simulink model "duc_model"  (R2023b)
settings: Solver=VariableStepDiscrete  StartTime=0.0  StopTime=DUC_LINEUP_param.endTime  RelTol=1e-3  EnableMultiTasking=on
PreLoadFcn:
  | % Run the setup script when the model is opened
  | setup_duc_model;
InitFcn:
  | % Run the setup script again just before the
  | % model is run, so that any updates made
  | % after opening are applied.
  | 
  | setup_duc_model;
StopFcn:
  | DUC_Output_analysis
values from neighbouring files (symbols this model uses):
  DUC_CM_multiplication_factor = 1    [setup_duc_model.m]
  DUC_CM_NCO_phase = [0 0 0 0]    [setup_duc_model.m]
  DUC_CM_NCO_sync = [0 0 0 0]    [setup_duc_model.m]
  DUC_CM_number_of_bits_to_shift_left = 0    [setup_duc_model.m]
undefined symbols (not defined in the file or in its folder): AdvDSPBChannelOutDisplay, dspba_ChannelInVis, dspba_ChannelOutVis, dspba_internal_get_channel_ports, DUC_LINEUP_param, latency, value
libraries: DSPBABase x17, DSPBAPrim x14, DSPBAFilters x6, simulink x4, DSPBAWaveformSynth x2, DSPBAModelBus x2
Description:
  | DSP Builder Advanced Template for Template Design implementing ModelIP designs
settings Model: Creator=mjervis  LastModifiedBy=5g
settings SolverCC: AlgebraicLoopSolver=TrustRegion
settings DataIOCC: LimitDataPoints=on  SaveFormat=Array  SignalLoggingSaveFormat=ModelDataLogs  ReturnWorkspaceOutputs=off
settings OptimizationCC: ExpressionDepthLimit=2147483647  LifeSpan=inf
settings DebuggingCC: UnderspecifiedInitializationDetection=Classic  MergeDetectMultiDrivingBlocksExec=none  SolverPrmCheckMsg=warning  InheritedTsInSrcMsg=none  IntegerOverflowMsg=none  FcnCallInpInsideContextMsg=warning  UnconnectedInputMsg=warning  UnconnectedOutputMsg=warning  UnconnectedLineMsg=warning  StateNameClashWarn=warning  SFUnexpectedBacktrackingDiag=warning  SFNoUnconditionalDefaultTransitionDiag=warning  SFExecutionAtInitializationDiag=none  IntegerSaturationMsg=none  ArithmeticOperatorsInVariantConditions=warning
settings HardwareCC: ProdBitPerPointer=32  ProdBitPerSizeT=32  ProdBitPerPtrDiffT=32  ProdLargestAtomicFloat=None  ProdIntDivRoundTo=Undefined  ProdEndianess=Unspecified  ProdWordSize=32  ProdHWDeviceType=32-bit Generic
settings ModelReferenceCC: EnableRefExpFcnMdlSchedulingChecks=on  PropagateSignalLabelsOutOfModel=off
settings SFSimCC: SimUseLocalCustomCode=off  CustomCodeUndefinedFunction=UseInterfaceOnly
settings RTWCC: RTWUseLocalCustomCode=off  DLArmComputeVersion=19.05
settings CodeAppCC: StateflowObjectComments=on
settings GRTTargetCC: TargetLangStandard=C89/C90 (ANSI)  CombineOutputUpdateFcns=off  GRTInterface=on
settings ConfigComp: CovMetricSettings=dw  CovSaveCumulativeToWorkspaceVar=on  CovSaveSingleToWorkspaceVar=on  CovExternalEMLEnable=off

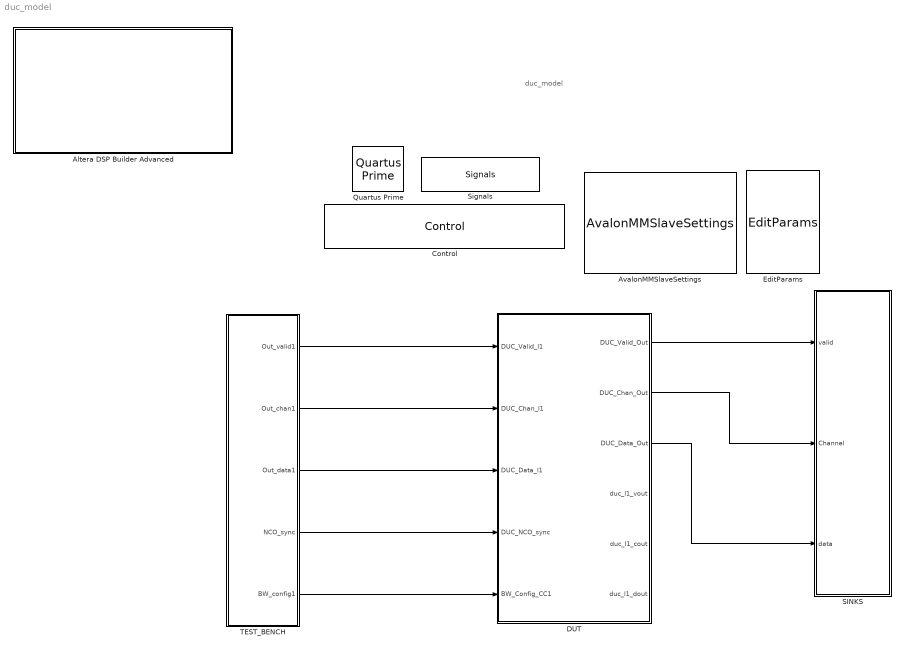
== system duc_model ==
  note: duc_model
  Altera DSP Builder Advanced : Subsystem  mask(DSP Builder Advanced Blockset Ignored Block){}
      settings: OpenFcn=web('http://www.altera.com', '-new');
      mask Display: image(imread('intellogo.tif'));
  AvalonMMSlaveSettings : DSPBABase/AvalonMMSlaveSettings
  Control : DSPBABase/Control  generate=on  language=VHDL  destination=./rtl  destination_gui=./rtl  make_full_path=off  path_is_relative=on  autotestbench=on  signaldepth=2  coveragetestbench=off  logs=off  spacewidth=2  spacenum=1  addrwidth=10  datawidth=16  dataendian=Big Endian  hierarchicalnames=off  ramThresholdBits=-1  distRamThresholdBits=-1  mlabThresholdBits=-1  hardMultiplierThresholdLuts=-1  version=20150801  errorOnChanMismatch=1  errorOnGPIOMismatch=0  importModelsimResults=0  cycleAccurate=off  reinterpretCastMult=off  paramFile=duc_model_params.xml
  DUT : Subsystem
  EditParams : DSPBABase/EditParams  version=20090407
  Quartus Prime : DSPBABase/Quartus Prime  version=20090407
  SINKS : Subsystem
  Signals : DSPBABase/Signals  clk=clk  freq=240  margin=0  rst=areset  rstactive=High  bus=bus  enbusclock=off  busfreq=491.52  bussync=off  version=20090407
  TEST_BENCH : Subsystem
  wires:
  DUT/1(DUC_Valid_Out) -> SINKS/1(valid)
  DUT/3(DUC_Data_Out) -> SINKS/3(data)
  DUT/2(DUC_Chan_Out) -> SINKS/2(Channel)
  TEST_BENCH/1(Out_valid1) -> DUT/1(DUC_Valid_l1)
  TEST_BENCH/2(Out_chan1) -> DUT/2(DUC_Chan_l1)
  TEST_BENCH/3(Out_data1) -> DUT/3(DUC_Data_l1)
  TEST_BENCH/4(NCO_sync) -> DUT/4(DUC_NCO_sync)
  TEST_BENCH/5(BW_config1) -> DUT/5(BW_Config_CC1)

== system duc_model/Altera DSP Builder Advanced ==

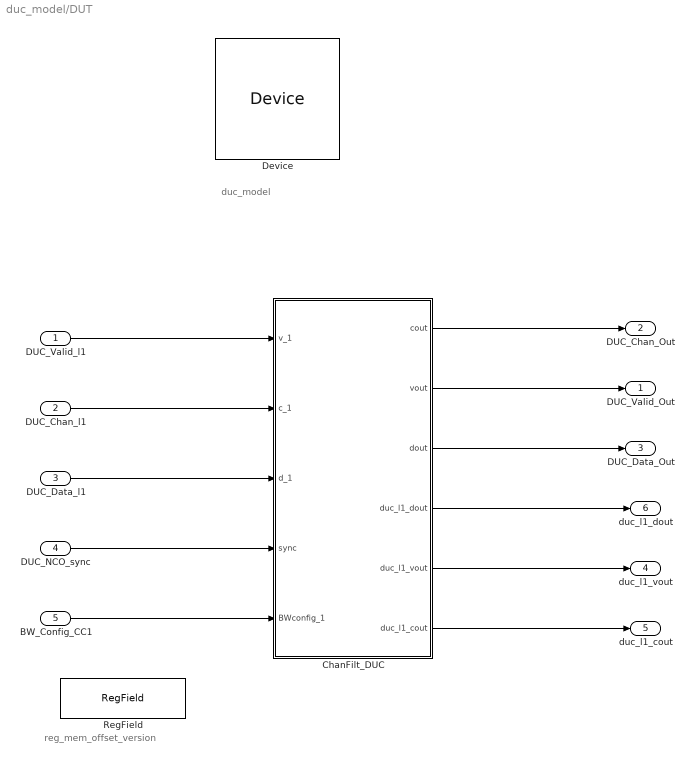
== system duc_model/DUT ==
  note: duc_model
  note: reg_mem_offset_version
  DUC_Valid_l1 : Inport
  DUC_Chan_l1 : Inport  Port=2
  DUC_Data_l1 : Inport  Port=3
  DUC_NCO_sync : Inport  Port=4
  BW_Config_CC1 : Inport  Port=5
  ChanFilt_DUC : Subsystem
  Device : DSPBABase/Device  family=Arria 10  deviceMember=Stratix V GX  stratix4device=Stratix IV GX  hardcopy4device=HardCopy IV E  stratix5device=Stratix V GX  device=10AS066N2F40I1SGES  speed=1  stratixSpeed=-5  stratix2Speed=-3  stratix3Speed=-3  stratix4gxSpeed=-2  stratix4gtSpeed=-1  cyclone2Speed=-6  cyclone3Speed=-7  arria2Speed=-4  cyclone4eSpeed=-8  stratix5Speed=-3  arria5Speed=-4  arriaSpeed=-6  cyclone3lsSpeed=-7  cyclone5Speed=-6  arria2gzSpeed=-3  nightFurySpeed=-2  ecp2Speed=-7  hardcopycompat=off  version=20140217  max10flashmode=off  max10nomeminit=off
  RegField : DSPBAModelBus/RegField  reg_name=DUC_LINEUP_param.reg_version.mem_offset  reg_rwmode=Read/Write  reg_msb=31  reg_lsb=0  reg_mode=Specify via dialog  reg_type=ufix(32)  reg_scale=2^0  reg_init=DUC_LINEUP_param.reg_version.Version_reg_val  reg_desc=Version_Output  reg_modal=off  reg_desc0=0  reg_desc1=0  reg_desc2=0  reg_desc3=0  reg_desc4=0  reg_desc5=0  reg_desc6=0  reg_desc7=0  reg_addr=808  SampleTime=-1  version=20090407
  DUC_Valid_Out : Outport
  DUC_Chan_Out : Outport  Port=2
  DUC_Data_Out : Outport  Port=3
  duc_l1_vout : Outport  Port=4
  duc_l1_cout : Outport  Port=5
  duc_l1_dout : Outport  Port=6
  wires:
  DUC_Valid_l1/1 -> ChanFilt_DUC/1(v_1)
  DUC_Chan_l1/1 -> ChanFilt_DUC/2(c_1)
  DUC_Data_l1/1 -> ChanFilt_DUC/3(d_1)
  ChanFilt_DUC/3(dout) -> DUC_Data_Out/1
  ChanFilt_DUC/2(vout) -> DUC_Valid_Out/1
  ChanFilt_DUC/1(cout) -> DUC_Chan_Out/1
  ChanFilt_DUC/5(duc_l1_vout) -> duc_l1_vout/1
  ChanFilt_DUC/6(duc_l1_cout) -> duc_l1_cout/1
  ChanFilt_DUC/4(duc_l1_dout) -> duc_l1_dout/1
  DUC_NCO_sync/1 -> ChanFilt_DUC/4(sync)
  BW_Config_CC1/1 -> ChanFilt_DUC/5(BWconfig_1)

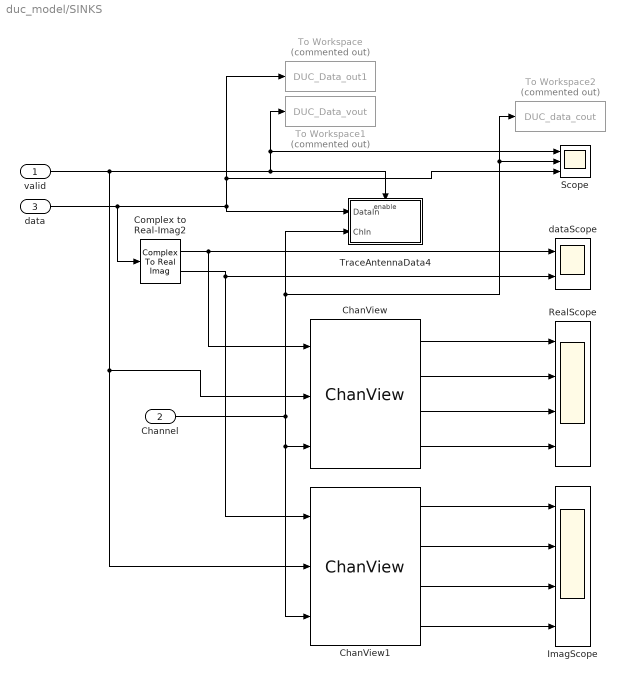
== system duc_model/SINKS ==
  valid : Inport
  Channel : Inport  Port=2
  data : Inport  Port=3
  ChanView : DSPBABase/ChanView  nchans=4  chan_vector=[0:3]  outsvalid=off  latency=1  version=20090407
  ChanView1 : DSPBABase/ChanView  nchans=4  chan_vector=[0:3]  outsvalid=off  latency=1  version=20090407
  Complex to Real-Imag2 : ComplexToRealImag
  ImagScope : Scope  NumInputPorts=4
  RealScope : Scope  NumInputPorts=4
  Scope : Scope  NumInputPorts=3
  To Workspace : ToWorkspace  Commented=on  VariableName=DUC_Data_out1  SampleTime=-1
  To Workspace1 : ToWorkspace  Commented=on  VariableName=DUC_Data_vout  SampleTime=-1
  To Workspace2 : ToWorkspace  Commented=on  VariableName=DUC_data_cout  SampleTime=-1
  TraceAntennaData4 : Subsystem  TreatAsAtomicUnit=on
  dataScope : Scope  NumInputPorts=2
  wires:
  valid/1 -> To Workspace1/1, Scope/1, TraceAntennaData4/Enable, ChanView1/2, ChanView/2
  data/1 -> TraceAntennaData4/1(DataIn), Scope/3, To Workspace/1, Complex to Real-Imag2/1
  Complex to Real-Imag2/1 -> ChanView/1, dataScope/1
  Channel/1 -> TraceAntennaData4/2(ChIn), To Workspace2/1, Scope/2, ChanView1/3, ChanView/3
  Complex to Real-Imag2/2 -> ChanView1/1, dataScope/2
  ChanView1/2 -> ImagScope/2
  ChanView1/3 -> ImagScope/3
  ChanView1/4 -> ImagScope/4
  ChanView1/1 -> ImagScope/1
  ChanView/3 -> RealScope/3
  ChanView/1 -> RealScope/1
  ChanView/4 -> RealScope/4
  ChanView/2 -> RealScope/2

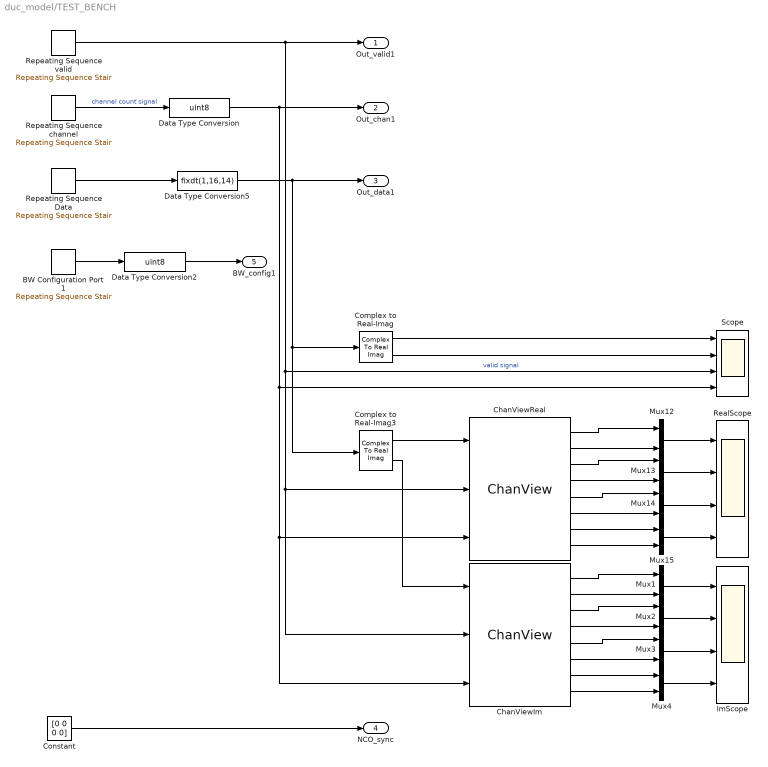
== system duc_model/TEST_BENCH ==
  BW Configuration Port 1 : simulink/Sources/Repeating Sequence Stair  OutValues=BW_Config_CC1  tsamp=1  OutMin=[]  OutMax=[]  OutDataTypeStr=fixdt(1,16)  OutputDataTypeScalingMode=Specify via dialog  OutDataType=fixdt(1,16)  ConRadixGroup=Best Precision: Vector-wise  OutScaling=[]
  ChanViewIm : DSPBABase/ChanView  nchans=8  chan_vector=[0:7]  outsvalid=off  latency=1  version=20090407
  ChanViewReal : DSPBABase/ChanView  nchans=8  chan_vector=[0:7]  outsvalid=off  latency=1  version=20090407
  Complex to Real-Imag : ComplexToRealImag
  Complex to Real-Imag3 : ComplexToRealImag
  Constant : Constant  Value=[0 0 0 0]  OutDataTypeStr=boolean
  Data Type Conversion : DataTypeConversion  OutDataTypeStr=uint8  SaturateOnIntegerOverflow=off  RndMeth=Floor
  Data Type Conversion2 : DataTypeConversion  OutDataTypeStr=uint8  SaturateOnIntegerOverflow=off  RndMeth=Floor
  Data Type Conversion5 : DataTypeConversion  OutDataTypeStr=fixdt(1,16,14)  SaturateOnIntegerOverflow=off  RndMeth=Floor
  ImScope : Scope  NumInputPorts=4
  Mux{1..4,12..15} (8 alike) : Mux  Inputs=2
  RealScope : Scope  NumInputPorts=4
  Repeating Sequence Data : simulink/Sources/Repeating Sequence Stair  OutValues=DUC_LINEUP_param.inputdata_l1  tsamp=1  OutMin=[]  OutMax=[]  OutDataTypeStr=fixdt(1,16)  OutputDataTypeScalingMode=Specify via dialog  OutDataType=fixdt(1,16)  ConRadixGroup=Best Precision: Vector-wise  OutScaling=[]
  Repeating Sequence channel : simulink/Sources/Repeating Sequence Stair  OutValues=DUC_LINEUP_param.duc_channel  tsamp=1  OutMin=[]  OutMax=[]  OutDataTypeStr=uint8  OutputDataTypeScalingMode=uint8  OutDataType=fixdt(1,16)  ConRadixGroup=Best Precision: Vector-wise  OutScaling=[]
  Repeating Sequence valid : simulink/Sources/Repeating Sequence Stair  OutValues=DUC_LINEUP_param.duc_valid  tsamp=1  OutMin=[]  OutMax=[]  OutDataTypeStr=fixdt('boolean')  OutputDataTypeScalingMode=Specify via dialog  OutDataType=fixdt('boolean')  ConRadixGroup=Best Precision: Vector-wise  OutScaling=[]
  Scope : Scope  NumInputPorts=4
  Out_valid1 : Outport
  Out_chan1 : Outport  Port=2
  Out_data1 : Outport  Port=3
  NCO_sync : Outport  Port=4
  BW_config1 : Outport  Port=5
  wires:
  Repeating Sequence Data/1 -> Data Type Conversion5/1
  Complex to Real-Imag/1 -> Scope/1
  Repeating Sequence valid/1 -> ChanViewIm/2, ChanViewReal/2, Scope/3, Out_valid1/1  "valid signal"
  Repeating Sequence channel/1 -> Data Type Conversion/1  "channel count signal"
  Data Type Conversion/1 -> ChanViewIm/3, ChanViewReal/3, Scope/4, Out_chan1/1
  Complex to Real-Imag/2 -> Scope/2
  Mux12/1 -> RealScope/1
  Mux13/1 -> RealScope/2
  Mux14/1 -> RealScope/3
  Mux15/1 -> RealScope/4
  Complex to Real-Imag3/1 -> ChanViewReal/1
  Complex to Real-Imag3/2 -> ChanViewIm/1
  ChanViewReal/1 -> Mux12/1
  ChanViewReal/2 -> Mux12/2
  ChanViewReal/3 -> Mux13/1
  ChanViewReal/4 -> Mux13/2
  ChanViewReal/5 -> Mux14/1
  ChanViewReal/6 -> Mux14/2
  ChanViewReal/7 -> Mux15/1
  ChanViewReal/8 -> Mux15/2
  ChanViewIm/1 -> Mux1/1
  ChanViewIm/7 -> Mux4/1
  ChanViewIm/8 -> Mux4/2
  Mux3/1 -> ImScope/3
  Mux4/1 -> ImScope/4
  Mux2/1 -> ImScope/2
  ChanViewIm/2 -> Mux1/2
  ChanViewIm/6 -> Mux3/2
  ChanViewIm/5 -> Mux3/1
  ChanViewIm/4 -> Mux2/2
  Mux1/1 -> ImScope/1
  ChanViewIm/3 -> Mux2/1
  Data Type Conversion5/1 -> Out_data1/1, Complex to Real-Imag/1, Complex to Real-Imag3/1
  Constant/1 -> NCO_sync/1
  BW Configuration Port 1/1 -> Data Type Conversion2/1
  Data Type Conversion2/1 -> BW_config1/1

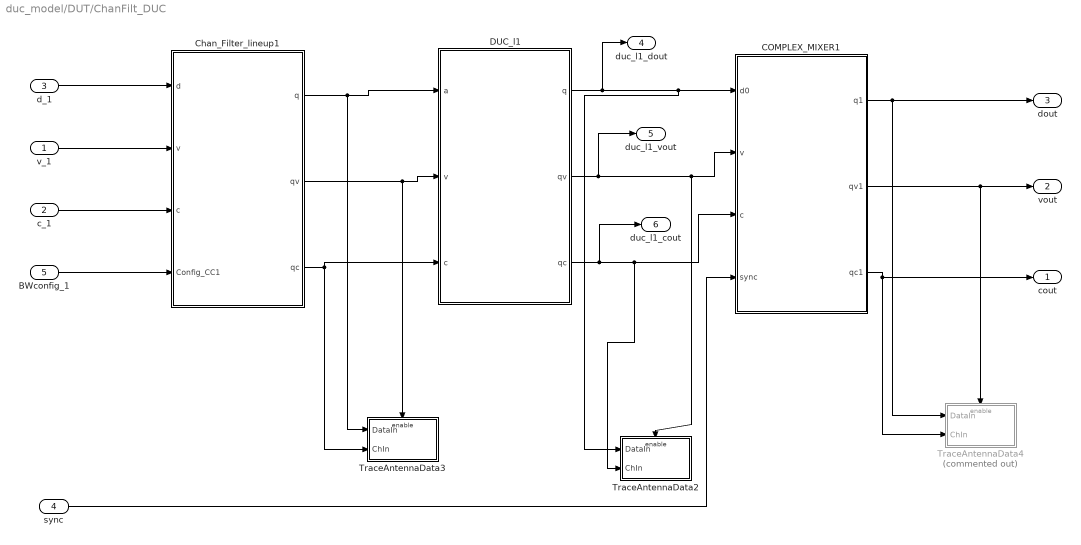
== system duc_model/DUT/ChanFilt_DUC ==
  v_1 : Inport
  c_1 : Inport  Port=2
  d_1 : Inport  Port=3
  sync : Inport  Port=4
  BWconfig_1 : Inport  Port=5
  COMPLEX_MIXER1 : Subsystem  mask{CM_clock_margin=DUC_LINEUP_param.ClockMargin, CM_pipeline_stages=DUC_LINEUP_param.NCO1.latency, CM_NCO_sample_rate=DUC_LINEUP_param.NCO1.sample_rate, CM_NCO_accumulator_bit_width=DUC_LINEUP_param.NCO1.accum_bit_width, CM_NCO_frequency_word=DUC_LINEUP_param.NCO1.freq_word, CM_NCO_base_addr=DUC_LINEUP_param.NCO1.base_addr, CM_NCO_data_type=DUC_LINEUP_param.NCO1.data_type, CM_NCO_scaling_value=DUC_LINEUP_param.NCO1.scaling_value, CM_sample_rate=DUC_LINEUP_param.CM.SampleRate, CM_complex_channels=DUC_LINEUP_param.CM.num_complex_chans, CM_complex_freq=DUC_LINEUP_param.CM.num_complex_freqs, CM_output_word_length=DUC_LINEUP_param.output_word_length, CM_output_fraction_length=DUC_LINEUP_param.output_fraction_length, CM_scale_multiplication_factor=DUC_CM_multiplication_factor, CM_scale_left_shift_factor=DUC_CM_number_of_bits_to_shift_left, CM_NCO_phase=DUC_CM_NCO_phase, CM_NCO_sync=DUC_CM_NCO_sync}
      mask prompts: CM_clock_margin "Clock margin"; CM_NCO_sample_rate "NCO sample rate"; CM_NCO_accumulator_bit_width "NCO accumulator bit width"; CM_NCO_frequency_word "NCO Frequency word"; CM_NCO_base_addr "NCO base address"; CM_NCO_data_type "NCO data type"; CM_NCO_scaling_value "NCO scaling value"; CM_sample_rate "Sample Rate"; CM_complex_channels "Number of complex channels"; CM_complex_freq "Number of complex frequencies"; CM_output_word_length "Output word length"; CM_output_fraction_length "Output fraction length"; CM_scale_multiplication_factor "Scale multiplication factor"; CM_scale_left_shift_factor "Scale left-shift factor"; CM_NCO_phase "NCO phase"; CM_NCO_sync "NCO sync"
      mask Display:
      | disp('COMPLEX\nMIXER');
      | port_label('input',1,'d');
      | port_label('input',2,'v');
      | port_label('input',3,'c');
      | port_label('input',4,'sync');
      | 
      | 
      | port_label('output',1,'q');
      | port_label('output',2,'qv');
      | port_label('output',3,'qc');
  Chan_Filter_lineup1 : Subsystem  mask{Clock_Margin=DUC_LINEUP_param.ClockMargin, NR_chan_filter_base_addr_l1_re=DUC_LINEUP_param.NR_chan_filter_100.chan_filt_base_addr_l1_re, NR_chan_filter_base_addr_l1_im=DUC_LINEUP_param.NR_chan_filter_100.chan_filt_base_addr_l1_im, NR_chan_filter_SampleRate=DUC_LINEUP_param.NR_chan_filter_100.Samplerate, NR_chan_filter_ChanCount=DUC_LINEUP_param.NR_chan_filter_100.ChanCount, ChannelFilter_coeffs=DUC_LINEUP_param.chan_filter.coeffs, CH_Multiplication_fact=1, CH_Bits_to_Left_shift=0, output_word_length=DUC_LINEUP_param.output_word_length, output_fraction_length=DUC_LINEUP_param.output_fraction_length}
      mask Display:
      | disp('DUC lineup');
      | port_label('input',1,'d');
      | port_label('input',2,'v');
      | port_label('input',3,'c');
      | 
      | port_label('output',1,'q');
      | port_label('output',2,'qv');
      | port_label('output',3,'qc');
  DUC_l1 : Subsystem
  TraceAntennaData2 : Subsystem  TreatAsAtomicUnit=on
  TraceAntennaData3 : Subsystem  TreatAsAtomicUnit=on
  TraceAntennaData4 : Subsystem  Commented=on  TreatAsAtomicUnit=on
  cout : Outport
  vout : Outport  Port=2
  dout : Outport  Port=3
  duc_l1_dout : Outport  Port=4
  duc_l1_vout : Outport  Port=5
  duc_l1_cout : Outport  Port=6
  wires:
  c_1/1 -> Chan_Filter_lineup1/3(c)
  d_1/1 -> Chan_Filter_lineup1/1(d)
  v_1/1 -> Chan_Filter_lineup1/2(v)
  Chan_Filter_lineup1/1(q) -> DUC_l1/1(a), TraceAntennaData3/1(DataIn)
  Chan_Filter_lineup1/2(qv) -> DUC_l1/2(v), TraceAntennaData3/Enable
  Chan_Filter_lineup1/3(qc) -> DUC_l1/3(c), TraceAntennaData3/2(ChIn)
  DUC_l1/3(qc) -> duc_l1_cout/1, COMPLEX_MIXER1/3(c), TraceAntennaData2/2(ChIn)
  DUC_l1/2(qv) -> duc_l1_vout/1, COMPLEX_MIXER1/2(v), TraceAntennaData2/Enable
  DUC_l1/1(q) -> duc_l1_dout/1, TraceAntennaData2/1(DataIn), COMPLEX_MIXER1/1(d0)
  COMPLEX_MIXER1/3(qc1) -> cout/1, TraceAntennaData4/2(ChIn)
  COMPLEX_MIXER1/2(qv1) -> vout/1, TraceAntennaData4/Enable
  COMPLEX_MIXER1/1(q1) -> dout/1, TraceAntennaData4/1(DataIn)
  sync/1 -> COMPLEX_MIXER1/4(sync)
  BWconfig_1/1 -> Chan_Filter_lineup1/4(Config_CC1)

== system duc_model/SINKS/TraceAntennaData4 ==
  DataIn : Inport
  ChIn : Inport  Port=2
  Enable : EnablePort
  DucAntDataOut : ToWorkspace  VariableName=Mixer_dOut  SampleTime=-1
  DucAntDataOut1 : ToWorkspace  VariableName=Mixer_cOut  SampleTime=-1
  wires:
  ChIn/1 -> DucAntDataOut1/1
  DataIn/1 -> DucAntDataOut/1

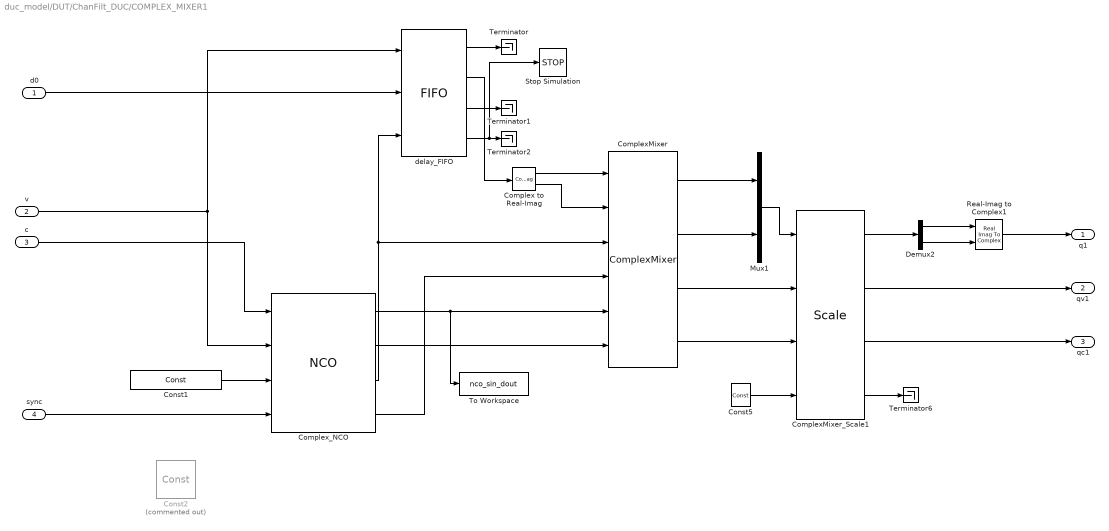
== system duc_model/DUT/ChanFilt_DUC/COMPLEX_MIXER1 ==
  d0 : Inport
  v : Inport  Port=2
  c : Inport  Port=3
  sync : Inport  Port=4
  Complex to Real-Imag : ComplexToRealImag
  ComplexMixer : DSPBAWaveformSynth/ComplexMixer  nInputRate=CM_sample_rate  nchan=CM_complex_channels  nfreq=CM_complex_freq  latency=5  simulationMode=Use Global Value  version=20090407
  ComplexMixer_Scale1 : DSPBABase/Scale  otype=sfix(CM_output_word_length)  scale=2^-CM_output_fraction_length  rndmethod=Biased  factor=CM_scale_multiplication_factor  satmethod=None  shift_vec=CM_scale_left_shift_factor  latency=1  simulationMode=Use Global Value  version=20130807
  Complex_NCO : DSPBAWaveformSynth/NCO  outputRate=CM_NCO_sample_rate  otype=sfix(CM_NCO_data_type)  scale=2^-CM_NCO_scaling_value  accumBitWidth=CM_NCO_accumulator_bit_width  phaseIncrAndInv=CM_NCO_frequency_word  phaseIncrAndInvMap=CM_NCO_base_addr  rwmode=Read/Write  exposebus=off  version=20090407  SampleTime=-1  expSFDR=96.32  accumPrecision=+/- 0.05722  phaseIncrInMHz="[50  1033.04       50  1033.04]"  outWidth=4  tableSize=8  latency=17
      settings: AttributesFormatString=%<latency>
  Const1 : DSPBAPrim/Const  primtype=const  nInputs=0  nOutputs=1  omode=Specify via dialog  otype=ufix(32)  scale=2^-0  rndmethod=Unbiased  factor=1  satmethod=Symmetric  shift_vec=[0 1 2 -1]  value=CM_NCO_phase  inPortNames=['+'; '+';]  outPortNames=[' ']  dspbaimage=dspba_prim.svg  text=fprintf('%s', num2str(value));  style=Optimised  visibilities=8 + 1024  floatPrecision=float32_m23  warnSaturation=on  version=20211007  SampleTime=inf
  Const2 : DSPBAPrim/Const  Commented=on  primtype=const  nInputs=0  nOutputs=1  omode=boolean  otype=sfix(16)  scale=2^-15  rndmethod=Unbiased  factor=1  satmethod=Symmetric  shift_vec=[0 1 2 -1]  value=[0 0 0 0]  inPortNames=['+'; '+';]  outPortNames=[' ']  dspbaimage=dspba_prim.svg  text=fprintf('%s', num2str(value));  style=Optimised  visibilities=8 + 1024  floatPrecision=float32_m23  warnSaturation=on  version=20211007  SampleTime=inf
  Const5 : DSPBAPrim/Const  primtype=const  nInputs=0  nOutputs=1  omode=Specify via dialog  otype=ufix(1)  scale=1  rndmethod=Unbiased  factor=1  satmethod=Symmetric  shift_vec=[0 1 2 -1]  value=0  inPortNames=['+'; '+';]  outPortNames=[' ']  dspbaimage=dspba_prim.svg  text=fprintf('%s', num2str(value));  style=Optimised  visibilities=8 + 1024  floatPrecision=float32_m23  warnSaturation=on  version=20211007  SampleTime=inf
  Demux2 : Demux  Outputs=2
  Mux1 : Mux  Inputs=2
  Real-Imag to Complex1 : RealImagToComplex
  Stop Simulation : Stop
  Terminator{,1..2,6} (4 alike) : Terminator
  To Workspace : ToWorkspace  VariableName=nco_sin_dout  SampleTime=-1
      settings: Save2DSignal=2-D array (concatenate along first dimension)
  delay_FIFO : DSPBAPrim/FIFO  primtype=fifo  nInputs=3  nOutputs=4  omode=Inherit via internal rule  otype=sfix(16)  scale=2^-15  rndmethod=Unbiased  factor=1  satmethod=Symmetric  shift_vec=[0 1 2 -1]  value=[64 4 63]  inPortNames=['w'; 'd'; 'r'; 'f']  outPortNames=['v'; 'q'; 't'; 'f']  dspbaimage=dspba_prim_tall.svg  text=fprintf('fifo');  style=Optimised  visibilities=263168  version=20211007  user_sclr=off
  q1 : Outport
  qv1 : Outport  Port=2
  qc1 : Outport  Port=3
  wires:
  Complex to Real-Imag/1 -> ComplexMixer/1
  Complex_NCO/3 -> ComplexMixer/3, delay_FIFO/3
  Demux2/2 -> Real-Imag to Complex1/2
  Complex_NCO/4 -> ComplexMixer/4
  Demux2/1 -> Real-Imag to Complex1/1
  v/1 -> delay_FIFO/1, Complex_NCO/2
  Complex_NCO/2 -> ComplexMixer/6
  delay_FIFO/3 -> Terminator1/1
  Mux1/1 -> ComplexMixer_Scale1/1
  delay_FIFO/2 -> Complex to Real-Imag/1
  ComplexMixer/4 -> ComplexMixer_Scale1/3
  d0/1 -> delay_FIFO/2
  Const5/1 -> ComplexMixer_Scale1/4
  delay_FIFO/4 -> Stop Simulation/1, Terminator2/1
  ComplexMixer/3 -> ComplexMixer_Scale1/2
  ComplexMixer/1 -> Mux1/1
  Complex_NCO/1 -> To Workspace/1, ComplexMixer/5
  ComplexMixer_Scale1/4 -> Terminator6/1
  ComplexMixer/2 -> Mux1/2
  ComplexMixer_Scale1/1 -> Demux2/1
  Const1/1 -> Complex_NCO/3
  Complex to Real-Imag/2 -> ComplexMixer/2
  delay_FIFO/1 -> Terminator/1
  c/1 -> Complex_NCO/1
  sync/1 -> Complex_NCO/4
  ComplexMixer_Scale1/3 -> qc1/1
  ComplexMixer_Scale1/2 -> qv1/1
  Real-Imag to Complex1/1 -> q1/1

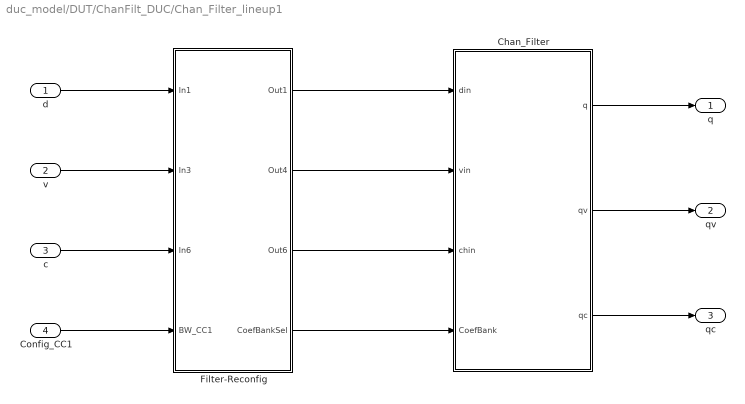
== system duc_model/DUT/ChanFilt_DUC/Chan_Filter_lineup1 ==
  d : Inport
  v : Inport  Port=2
  c : Inport  Port=3
  Config_CC1 : Inport  Port=4
  Chan_Filter : Subsystem
  Filter-Reconfig : Subsystem
  q : Outport
  qv : Outport  Port=2
  qc : Outport  Port=3
  wires:
  Chan_Filter/3(qc) -> qc/1
  Chan_Filter/2(qv) -> qv/1
  Chan_Filter/1(q) -> q/1
  d/1 -> Filter-Reconfig/1(In1)
  v/1 -> Filter-Reconfig/2(In3)
  c/1 -> Filter-Reconfig/3(In6)
  Filter-Reconfig/1(Out1) -> Chan_Filter/1(din)
  Filter-Reconfig/2(Out4) -> Chan_Filter/2(vin)
  Filter-Reconfig/3(Out6) -> Chan_Filter/3(chin)
  Filter-Reconfig/4(CoefBankSel) -> Chan_Filter/4(CoefBank)
  Config_CC1/1 -> Filter-Reconfig/4(BW_CC1)

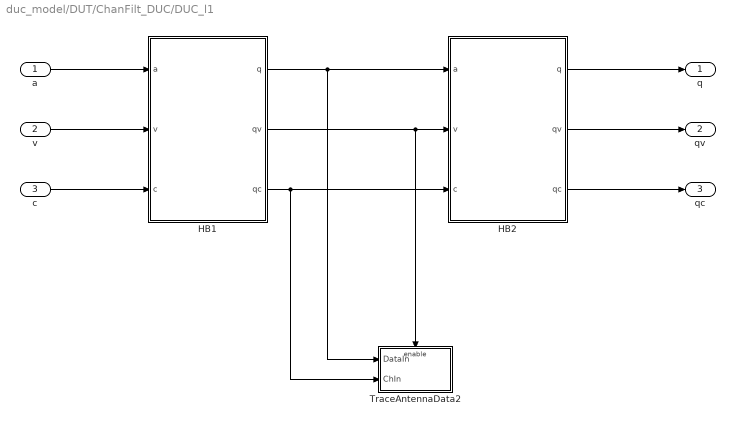
== system duc_model/DUT/ChanFilt_DUC/DUC_l1 ==
  a : Inport
  v : Inport  Port=2
  c : Inport  Port=3
  HB1 : Subsystem
  HB2 : Subsystem
  TraceAntennaData2 : Subsystem  TreatAsAtomicUnit=on
  q : Outport
  qv : Outport  Port=2
  qc : Outport  Port=3
  wires:
  a/1 -> HB1/1(a)
  v/1 -> HB1/2(v)
  c/1 -> HB1/3(c)
  HB2/1(q) -> q/1
  HB2/2(qv) -> qv/1
  HB2/3(qc) -> qc/1
  HB1/1(q) -> TraceAntennaData2/1(DataIn), HB2/1(a)
  HB1/2(qv) -> HB2/2(v), TraceAntennaData2/Enable
  HB1/3(qc) -> TraceAntennaData2/2(ChIn), HB2/3(c)

== system duc_model/DUT/ChanFilt_DUC/TraceAntennaData2 ==
  DataIn : Inport
  ChIn : Inport  Port=2
  Enable : EnablePort
  DucAntDataOut : ToWorkspace  VariableName=Mixer_dIn  SampleTime=-1
  DucAntDataOut1 : ToWorkspace  VariableName=Mixer_cIn  SampleTime=-1
  wires:
  DataIn/1 -> DucAntDataOut/1
  ChIn/1 -> DucAntDataOut1/1

== system duc_model/DUT/ChanFilt_DUC/TraceAntennaData3 ==
  DataIn : Inport
  ChIn : Inport  Port=2
  Enable : EnablePort
  DucAntDataOut : ToWorkspace  VariableName=chFilt_dOut  SampleTime=-1
  DucAntDataOut1 : ToWorkspace  VariableName=chFilt_cOut  SampleTime=-1
  wires:
  ChIn/1 -> DucAntDataOut1/1
  DataIn/1 -> DucAntDataOut/1

== system duc_model/DUT/ChanFilt_DUC/TraceAntennaData4 ==
  DataIn : Inport
  ChIn : Inport  Port=2
  Enable : EnablePort
  DucAntDataOut : ToWorkspace  VariableName=Mixer_dOut  SampleTime=-1
  DucAntDataOut1 : ToWorkspace  VariableName=Mixer_cOut  SampleTime=-1
  wires:
  ChIn/1 -> DucAntDataOut1/1
  DataIn/1 -> DucAntDataOut/1

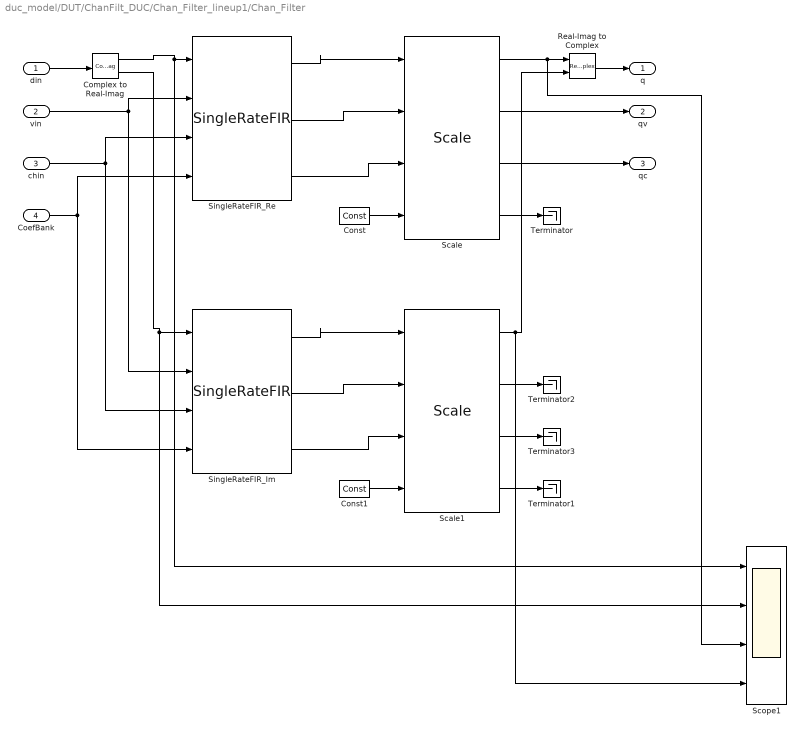
== system duc_model/DUT/ChanFilt_DUC/Chan_Filter_lineup1/Chan_Filter ==
  din : Inport
  vin : Inport  Port=2
  chin : Inport  Port=3
  CoefBank : Inport  Port=4
  Complex to Real-Imag : ComplexToRealImag
  Const : DSPBAPrim/Const  primtype=const  nInputs=0  nOutputs=1  omode=Specify via dialog  otype=uint(1)  scale=2^0  rndmethod=Unbiased  factor=1  satmethod=Symmetric  shift_vec=[0 1 2 -1]  value=0  inPortNames=['+'; '+';]  outPortNames=[' ']  dspbaimage=dspba_prim.svg  text=fprintf('%s', num2str(value));  style=Optimised  visibilities=8 + 1024  floatPrecision=float32_m23  warnSaturation=on  version=20211007  SampleTime=inf
  Const1 : DSPBAPrim/Const  primtype=const  nInputs=0  nOutputs=1  omode=Specify via dialog  otype=uint(1)  scale=2^0  rndmethod=Unbiased  factor=1  satmethod=Symmetric  shift_vec=[0 1 2 -1]  value=0  inPortNames=['+'; '+';]  outPortNames=[' ']  dspbaimage=dspba_prim.svg  text=fprintf('%s', num2str(value));  style=Optimised  visibilities=8 + 1024  floatPrecision=float32_m23  warnSaturation=on  version=20211007  SampleTime=inf
  Real-Imag to Complex : RealImagToComplex
  Scale : DSPBABase/Scale  otype=sfix(output_word_length)  scale=2^-(output_fraction_length)  rndmethod=Biased  factor=CH_Multiplication_fact  satmethod=None  shift_vec=CH_Bits_to_Left_shift  latency=2  simulationMode=Use Global Value  version=20130807
      settings: AttributesFormatString=%<latency>
  Scale1 : DSPBABase/Scale  otype=sfix(output_word_length)  scale=2^-(output_fraction_length)  rndmethod=Biased  factor=CH_Multiplication_fact  satmethod=None  shift_vec=CH_Bits_to_Left_shift  latency=2  simulationMode=Use Global Value  version=20130807
      settings: AttributesFormatString=%<latency>
  Scope1 : Scope  NumInputPorts=4
  SingleRateFIR_Im : DSPBAFilters/SingleRateFIR  nInputRate=NR_chan_filter_SampleRate  nchan=NR_chan_filter_ChanCount  symmetry=Symmetrical  coef=ChannelFilter_coeffs  addr=NR_chan_filter_base_addr_l1_im  rwmode=Read/Write  nband=Use All Taps  latency=71  exposebus=off  version=20090407  recon=off  MM=[0,1,2,3,4,5,6,7,8,9,10,11,12,13,14,15,16,17,18,19]  resetrezero=off  sharecoef=auto  simulationMode=Standard
      settings: AttributesFormatString=%<latency>
  SingleRateFIR_Re : DSPBAFilters/SingleRateFIR  nInputRate=NR_chan_filter_SampleRate  nchan=NR_chan_filter_ChanCount  symmetry=Symmetrical  coef=ChannelFilter_coeffs  addr=NR_chan_filter_base_addr_l1_re  rwmode=Read/Write  nband=Use All Taps  latency=71  exposebus=off  version=20090407  recon=off  MM=[0,1,2,3,4,5,6,7,8,9,10,11,12,13,14,15,16,17,18,19]  resetrezero=off  sharecoef=auto  simulationMode=Standard
      settings: AttributesFormatString=%<latency>
  Terminator{,1..3} (4 alike) : Terminator
  q : Outport
  qv : Outport  Port=2
  qc : Outport  Port=3
  wires:
  SingleRateFIR_Re/1 -> Scale/1
  SingleRateFIR_Re/2 -> Scale/2
  SingleRateFIR_Re/3 -> Scale/3
  Scale/4 -> Terminator/1
  Const/1 -> Scale/4
  vin/1 -> SingleRateFIR_Re/2, SingleRateFIR_Im/2
  chin/1 -> SingleRateFIR_Im/3, SingleRateFIR_Re/3
  Scale/2 -> qv/1
  Scale/3 -> qc/1
  Scale/1 -> Scope1/3, Real-Imag to Complex/1
  Scale1/4 -> Terminator1/1
  Const1/1 -> Scale1/4
  SingleRateFIR_Im/1 -> Scale1/1
  SingleRateFIR_Im/3 -> Scale1/3
  Scale1/1 -> Scope1/4, Real-Imag to Complex/2
  SingleRateFIR_Im/2 -> Scale1/2
  Complex to Real-Imag/1 -> Scope1/1, SingleRateFIR_Re/1
  din/1 -> Complex to Real-Imag/1
  Complex to Real-Imag/2 -> Scope1/2, SingleRateFIR_Im/1
  Real-Imag to Complex/1 -> q/1
  Scale1/2 -> Terminator2/1
  Scale1/3 -> Terminator3/1
  CoefBank/1 -> SingleRateFIR_Im/4, SingleRateFIR_Re/4

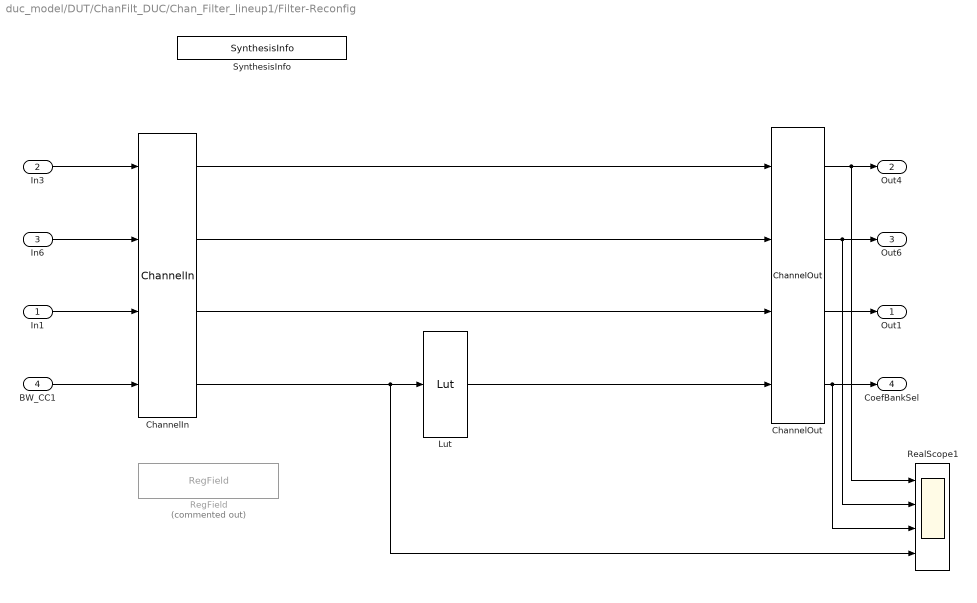
== system duc_model/DUT/ChanFilt_DUC/Chan_Filter_lineup1/Filter-Reconfig ==
  In1 : Inport
  In3 : Inport  Port=2
  In6 : Inport  Port=3
  BW_CC1 : Inport  Port=4
  ChannelIn : DSPBAPrim/ChannelIn  primtype=channelin  nInputs=dspba_internal_get_channel_ports(gcb)  nOutputs=dspba_internal_get_channel_ports(gcb)  omode=Inherit via internal rule  otype=sfix(16)  scale=2^-15  rndmethod=Unbiased  factor=1  satmethod=Symmetric  shift_vec=[0 1 2 -1]  value=2  inPortNames=['v'; 'c'; '0'; '1'; '2'; '3'; '4'; '5'; '6'; '7'; '8'; '9'; 'A'; 'B'; 'D'; 'E'; 'F'; 'G'; 'H'; 'I'; 'J'; 'K'; 'L'; 'M'; 'N'; 'O'; 'P'; 'Q'; 'R'; 'S'; 'T'; 'U'; 'W'; 'X'; 'Y'; 'Z']  outPortNames=['v'; 'c'; '0'; '1'; '2'; '3'; '4'; '5'; '6'; '7'; '8'; '9'; 'A'; 'B'; 'D'; 'E'; 'F'; 'G'; 'H'; 'I'; 'J'; 'K'; 'L'; 'M'; 'N'; 'O'; 'P'; 'Q'; 'R'; 'S'; 'T'; 'U'; 'W'; 'X'; 'Y'; 'Z']  dspbaimage=dspba_prim_channel_tall.svg  text=fprintf('In');  style=Optimised  dataSignals=2  foldingEnabled=off  channels=1  sampleRate=200  packetBeginPresent=off  packetBeginEnabled=off  visibilities=dspba_ChannelInVis(gcb)  scheduleOrigin=on  version=20211214
  ChannelOut : DSPBAPrim/ChannelOut  primtype=channelout  nInputs=dspba_internal_get_channel_ports(gcb)  nOutputs=dspba_internal_get_channel_ports(gcb)  omode=Inherit via internal rule  otype=sfix(16)  scale=2^-15  rndmethod=Unbiased  factor=1  satmethod=Symmetric  shift_vec=[0 1 2 -1]  value=2  inPortNames=['v'; 'c'; '0'; '1'; '2'; '3'; '4'; '5'; '6'; '7'; '8'; '9'; 'A'; 'B'; 'D'; 'E'; 'F'; 'G'; 'H'; 'I'; 'J'; 'K'; 'L'; 'M'; 'N'; 'O'; 'P'; 'Q'; 'R'; 'S'; 'T'; 'U'; 'W'; 'X'; 'Y'; 'Z']  outPortNames=['v'; 'c'; '0'; '1'; '2'; '3'; '4'; '5'; '6'; '7'; '8'; '9'; 'A'; 'B'; 'D'; 'E'; 'F'; 'G'; 'H'; 'I'; 'J'; 'K'; 'L'; 'M'; 'N'; 'O'; 'P'; 'Q'; 'R'; 'S'; 'T'; 'U'; 'W'; 'X'; 'Y'; 'Z']  dspbaimage=dspba_prim_channel_tall.svg  text=fprintf('Out%s', AdvDSPBChannelOutDisplay(latency));  style=Optimised  dataSignals=2  foldingEnabled=off  channels=1  sampleRate=200  packetBeginPresent=off  packetBeginEnabled=off  visibilities=dspba_ChannelOutVis(gcb)  latency=2  version=20211214
  Lut : DSPBAPrim/Lut  primtype=lut  nInputs=1  nOutputs=1  omode=Inherit via internal rule  otype=sfix(16)  scale=2^-15  rndmethod=Unbiased  factor=1  satmethod=Symmetric  shift_vec=[0 1 2 -1]  value=[0 0 0 0 0 0 0 0 0 0 0 0 0 0 1 zeros(1,241)]  inPortNames=[' '; ' ';]  outPortNames=[' ']  dspbaimage=dspba_prim.svg  text=fprintf('LUT');  style=Optimised  visibilities=8 + 1024  floatPrecision=float32_m23  version=20211007
  RealScope1 : Scope  NumInputPorts=4
  RegField : DSPBAModelBus/RegField  Commented=on  reg_name=BW_Config_CC1_Offset  reg_rwmode=Read/Write  reg_msb=7  reg_lsb=0  reg_mode=Specify via dialog  reg_type=ufix(8)  reg_scale=2^0  reg_init=BW_Config_CC1  reg_desc=BW Configuration Register for CC1  reg_modal=off  reg_desc0=0  reg_desc1=0  reg_desc2=0  reg_desc3=0  reg_desc4=0  reg_desc5=0  reg_desc6=0  reg_desc7=0  reg_addr=0  SampleTime=-1  version=20090407
  SynthesisInfo : DSPBAPrim/SynthesisInfo  primtype=synthinfo  nInputs=0  nOutputs=0  omode=Inherit via internal rule  otype=sfix(16)  scale=2^-15  rndmethod=Truncate  factor=1  satmethod=Symmetric  shift_vec=[0 1 2 -1]  value=99  inPortNames=[' '; ' ';]  outPortNames=[' ']  dspbaimage=dspba_prim_ctrl.jpg  text=fprintf('Style=%s', style);  style=Scheduled  visibilities=2^15+2^17+2^18+2^19  constraintPair=None  constraintRelation=>  constraintLimit=Latency  modelRefSign=+  modelRef=''  showSchedule=off  simulationMode=Use Global Value  resetMinimization=Conditional - On for ChannelIn/Out only  version=20220106
  Out1 : Outport
  Out4 : Outport  Port=2
  Out6 : Outport  Port=3
  CoefBankSel : Outport  Port=4
  wires:
  ChannelOut/2 -> RealScope1/2, Out6/1
  In3/1 -> ChannelIn/1
  In1/1 -> ChannelIn/3
  In6/1 -> ChannelIn/2
  ChannelOut/1 -> RealScope1/1, Out4/1
  ChannelOut/3 -> Out1/1
  ChannelOut/4 -> RealScope1/3, CoefBankSel/1
  Lut/1 -> ChannelOut/4
  ChannelIn/1 -> ChannelOut/1
  ChannelIn/2 -> ChannelOut/2
  ChannelIn/3 -> ChannelOut/3
  BW_CC1/1 -> ChannelIn/4
  ChannelIn/4 -> RealScope1/4, Lut/1

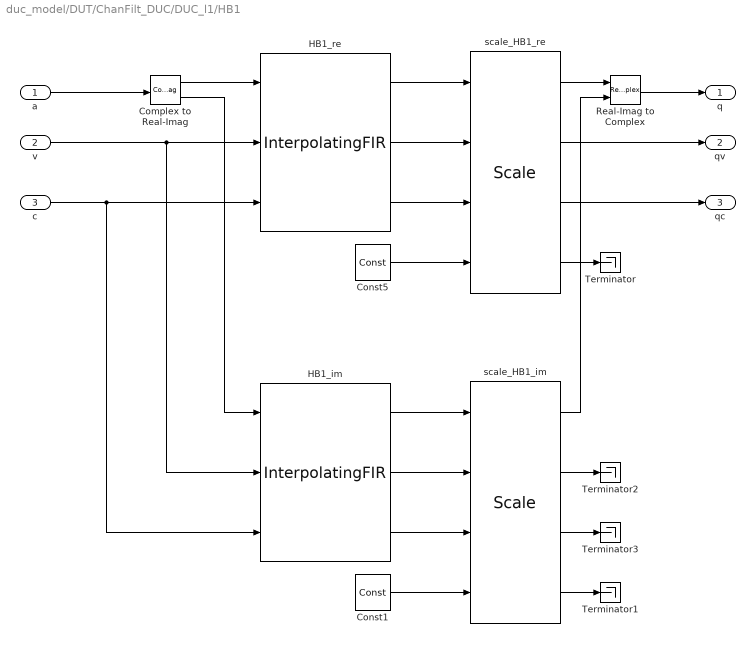
== system duc_model/DUT/ChanFilt_DUC/DUC_l1/HB1 ==
  a : Inport
  v : Inport  Port=2
  c : Inport  Port=3
  Complex to Real-Imag : ComplexToRealImag
  Const1 : DSPBAPrim/Const  primtype=const  nInputs=0  nOutputs=1  omode=Inherit via internal rule  otype=sfix(16)  scale=2^-15  rndmethod=Unbiased  factor=1  satmethod=Symmetric  shift_vec=[0 1 2 -1]  value=0  inPortNames=['+'; '+';]  outPortNames=[' ']  dspbaimage=dspba_prim.svg  text=fprintf('%s', num2str(value));  style=Optimised  visibilities=8 + 1024  floatPrecision=float32_m23  warnSaturation=on  version=20211007  SampleTime=inf
  Const5 : DSPBAPrim/Const  primtype=const  nInputs=0  nOutputs=1  omode=Inherit via internal rule  otype=sfix(16)  scale=2^-15  rndmethod=Unbiased  factor=1  satmethod=Symmetric  shift_vec=[0 1 2 -1]  value=0  inPortNames=['+'; '+';]  outPortNames=[' ']  dspbaimage=dspba_prim.svg  text=fprintf('%s', num2str(value));  style=Optimised  visibilities=8 + 1024  floatPrecision=float32_m23  warnSaturation=on  version=20211007  SampleTime=inf
  HB1_im : DSPBAFilters/InterpolatingFIR  nInputRate=DUC_LINEUP_param.HB_filt1.SampleRate  interp=DUC_LINEUP_param.HB_filt1.Interpolation  nchan=DUC_LINEUP_param.HB_filt1.ChanCount  symmetry=Symmetrical  coef=DUC_LINEUP_param.HB_filt1.coeffs  addr=DUC_LINEUP_param.HB_filt6.base_addr_l3  rwmode=Constant  nband=Half Band  exposebus=off  latency=9  version=20090407  recon=off  MM=[0,1,2,3,4,5,6,7,8,9,10,11,12,13,14,15]  resetrezero=off  sharecoef=auto  simulationMode=Standard
  HB1_re : DSPBAFilters/InterpolatingFIR  nInputRate=DUC_LINEUP_param.HB_filt1.SampleRate  interp=DUC_LINEUP_param.HB_filt1.Interpolation  nchan=DUC_LINEUP_param.HB_filt1.ChanCount  symmetry=Symmetrical  coef=DUC_LINEUP_param.HB_filt1.coeffs  addr=DUC_LINEUP_param.HB_filt6.base_addr_l3  rwmode=Constant  nband=Half Band  exposebus=off  latency=9  version=20090407  recon=off  MM=[0,1,2,3,4,5,6,7,8,9,10,11,12,13,14,15]  resetrezero=off  sharecoef=auto  simulationMode=Standard
  Real-Imag to Complex : RealImagToComplex
  Terminator{,1..3} (4 alike) : Terminator
  scale_HB1_im : DSPBABase/Scale  otype=sfix(DUC_LINEUP_param.output_word_length)  scale=2^-DUC_LINEUP_param.output_fraction_length  rndmethod=Biased  factor=1  satmethod=None  shift_vec=1  latency=2  simulationMode=Use Global Value  version=20090407
  scale_HB1_re : DSPBABase/Scale  otype=sfix(DUC_LINEUP_param.output_word_length)  scale=2^-DUC_LINEUP_param.output_fraction_length  rndmethod=Biased  factor=1  satmethod=None  shift_vec=1  latency=2  simulationMode=Use Global Value  version=20090407
  q : Outport
  qv : Outport  Port=2
  qc : Outport  Port=3
  wires:
  scale_HB1_im/4 -> Terminator1/1
  scale_HB1_re/4 -> Terminator/1
  Complex to Real-Imag/2 -> HB1_im/1
  a/1 -> Complex to Real-Imag/1
  scale_HB1_im/2 -> Terminator2/1
  Const1/1 -> scale_HB1_im/4
  HB1_re/1 -> scale_HB1_re/1
  scale_HB1_im/1 -> Real-Imag to Complex/2
  Complex to Real-Imag/1 -> HB1_re/1
  scale_HB1_re/2 -> qv/1
  HB1_re/2 -> scale_HB1_re/2
  Const5/1 -> scale_HB1_re/4
  HB1_im/1 -> scale_HB1_im/1
  HB1_im/3 -> scale_HB1_im/3
  c/1 -> HB1_im/3, HB1_re/3
  scale_HB1_im/3 -> Terminator3/1
  scale_HB1_re/3 -> qc/1
  v/1 -> HB1_im/2, HB1_re/2
  HB1_re/3 -> scale_HB1_re/3
  scale_HB1_re/1 -> Real-Imag to Complex/1
  Real-Imag to Complex/1 -> q/1
  HB1_im/2 -> scale_HB1_im/2

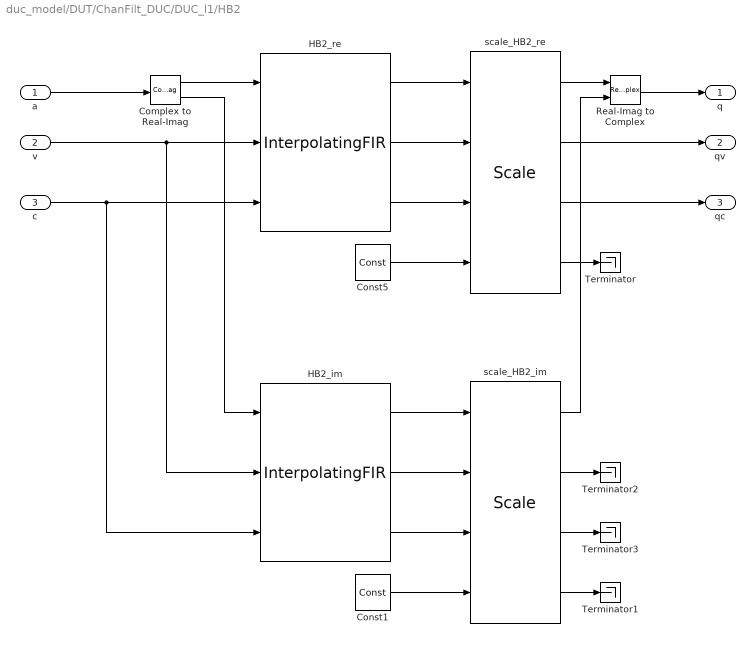
== system duc_model/DUT/ChanFilt_DUC/DUC_l1/HB2 ==
  a : Inport
  v : Inport  Port=2
  c : Inport  Port=3
  Complex to Real-Imag : ComplexToRealImag
  Const1 : DSPBAPrim/Const  primtype=const  nInputs=0  nOutputs=1  omode=Inherit via internal rule  otype=sfix(16)  scale=2^-15  rndmethod=Unbiased  factor=1  satmethod=Symmetric  shift_vec=[0 1 2 -1]  value=0  inPortNames=['+'; '+';]  outPortNames=[' ']  dspbaimage=dspba_prim.svg  text=fprintf('%s', num2str(value));  style=Optimised  visibilities=8 + 1024  floatPrecision=float32_m23  warnSaturation=on  version=20211007  SampleTime=inf
  Const5 : DSPBAPrim/Const  primtype=const  nInputs=0  nOutputs=1  omode=Inherit via internal rule  otype=sfix(16)  scale=2^-15  rndmethod=Unbiased  factor=1  satmethod=Symmetric  shift_vec=[0 1 2 -1]  value=0  inPortNames=['+'; '+';]  outPortNames=[' ']  dspbaimage=dspba_prim.svg  text=fprintf('%s', num2str(value));  style=Optimised  visibilities=8 + 1024  floatPrecision=float32_m23  warnSaturation=on  version=20211007  SampleTime=inf
  HB2_im : DSPBAFilters/InterpolatingFIR  nInputRate=DUC_LINEUP_param.HB_filt2.SampleRate  interp=DUC_LINEUP_param.HB_filt2.Interpolation  nchan=DUC_LINEUP_param.HB_filt2.ChanCount  symmetry=Symmetrical  coef=DUC_LINEUP_param.HB_filt2.coeffs  addr=DUC_LINEUP_param.HB_filt6.base_addr_l3  rwmode=Constant  nband=Half Band  exposebus=off  latency=7  version=20090407  recon=off  MM=[0,1,2,3,4,5,6,7,8,9,10,11,12,13,14,15]  resetrezero=off  sharecoef=auto  simulationMode=Standard
  HB2_re : DSPBAFilters/InterpolatingFIR  nInputRate=DUC_LINEUP_param.HB_filt2.SampleRate  interp=DUC_LINEUP_param.HB_filt2.Interpolation  nchan=DUC_LINEUP_param.HB_filt2.ChanCount  symmetry=Symmetrical  coef=DUC_LINEUP_param.HB_filt2.coeffs  addr=DUC_LINEUP_param.HB_filt6.base_addr_l3  rwmode=Constant  nband=Half Band  exposebus=off  latency=7  version=20090407  recon=off  MM=[0,1,2,3,4,5,6,7,8,9,10,11,12,13,14,15]  resetrezero=off  sharecoef=auto  simulationMode=Standard
  Real-Imag to Complex : RealImagToComplex
  Terminator{,1..3} (4 alike) : Terminator
  scale_HB2_im : DSPBABase/Scale  otype=sfix(DUC_LINEUP_param.output_word_length)  scale=2^-DUC_LINEUP_param.output_fraction_length  rndmethod=Biased  factor=1  satmethod=None  shift_vec=1  latency=2  simulationMode=Use Global Value  version=20090407
  scale_HB2_re : DSPBABase/Scale  otype=sfix(DUC_LINEUP_param.output_word_length)  scale=2^-DUC_LINEUP_param.output_fraction_length  rndmethod=Biased  factor=1  satmethod=None  shift_vec=1  latency=2  simulationMode=Use Global Value  version=20090407
  q : Outport
  qv : Outport  Port=2
  qc : Outport  Port=3
  wires:
  HB2_im/2 -> scale_HB2_im/2
  Real-Imag to Complex/1 -> q/1
  scale_HB2_re/1 -> Real-Imag to Complex/1
  HB2_re/3 -> scale_HB2_re/3
  v/1 -> HB2_im/2, HB2_re/2
  scale_HB2_re/3 -> qc/1
  scale_HB2_im/3 -> Terminator3/1
  c/1 -> HB2_im/3, HB2_re/3
  HB2_im/3 -> scale_HB2_im/3
  HB2_im/1 -> scale_HB2_im/1
  Const5/1 -> scale_HB2_re/4
  HB2_re/2 -> scale_HB2_re/2
  scale_HB2_re/2 -> qv/1
  Complex to Real-Imag/1 -> HB2_re/1
  scale_HB2_im/1 -> Real-Imag to Complex/2
  HB2_re/1 -> scale_HB2_re/1
  Const1/1 -> scale_HB2_im/4
  scale_HB2_im/2 -> Terminator2/1
  a/1 -> Complex to Real-Imag/1
  Complex to Real-Imag/2 -> HB2_im/1
  scale_HB2_re/4 -> Terminator/1
  scale_HB2_im/4 -> Terminator1/1

== system duc_model/DUT/ChanFilt_DUC/DUC_l1/TraceAntennaData2 ==
  DataIn : Inport
  ChIn : Inport  Port=2
  Enable : EnablePort
  DucAntDataOut : ToWorkspace  VariableName=HB1_dOut  SampleTime=-1
  DucAntDataOut1 : ToWorkspace  VariableName=HB1_cOut  SampleTime=-1
  wires:
  DataIn/1 -> DucAntDataOut/1
  ChIn/1 -> DucAntDataOut1/1
